simulink model "Pacemaker_Final_01"  (R2020a)
settings: Solver=FixedStepAuto  StartTime=0.0  StopTime=10.0  FixedStep=1e-3  RelTol=1e-3  EnableMultiTasking=on
undefined symbols (not defined in the file): D0, D1, D10, D11, D12, D13, D2, D3, D4, D5, D6, D7, D8, D9, PTA0, PTA1, PTA2, PTB23, PTB9, PTC16, PTC17, PTC2, PTC3, PTC4, PTD0, PTD1, PTD2, PTD3
libraries: frdmk64flib x20
settings Model: ExtModeTrigDuration=5  Creator=forre  LastModifiedBy=forre
settings OptimizationCC: EnhancedBackFolding=on  PassReuseOutputArgsAs=Individual arguments  ZeroExternalMemoryAtStartup=off  ZeroInternalMemoryAtStartup=off  MaxStackSize=64  OptimizeBlockOrder=speed  DifferentSizesBufferReuse=on  OptimizationCustomize=off  EfficientTunableParamExpr=on
settings DebuggingCC: ParameterTunabilityLossMsg=error
settings HardwareCC: ProdBitPerPointer=32  ProdBitPerSizeT=32  ProdBitPerPtrDiffT=32  ProdLargestAtomicInteger=Long  ProdLargestAtomicFloat=Double  ProdWordSize=32  ProdHWDeviceType=ARM Compatible->ARM Cortex
settings SFSimCC: MATLABDynamicMemAlloc=off
settings RTWCC: SystemTargetFile=ert.tlc  HardwareBoard=NXP FRDM-K64F  TemplateMakefile=ert_default_tmf  Toolchain=GNU Tools for ARM Embedded Processors
settings CodeAppCC: ForceParamTrailComments=on  IgnoreCustomStorageClasses=off  OperatorAnnotations=on  SimulinkDataObjDesc=on  SFDataObjDesc=on  InsertBlockDesc=on

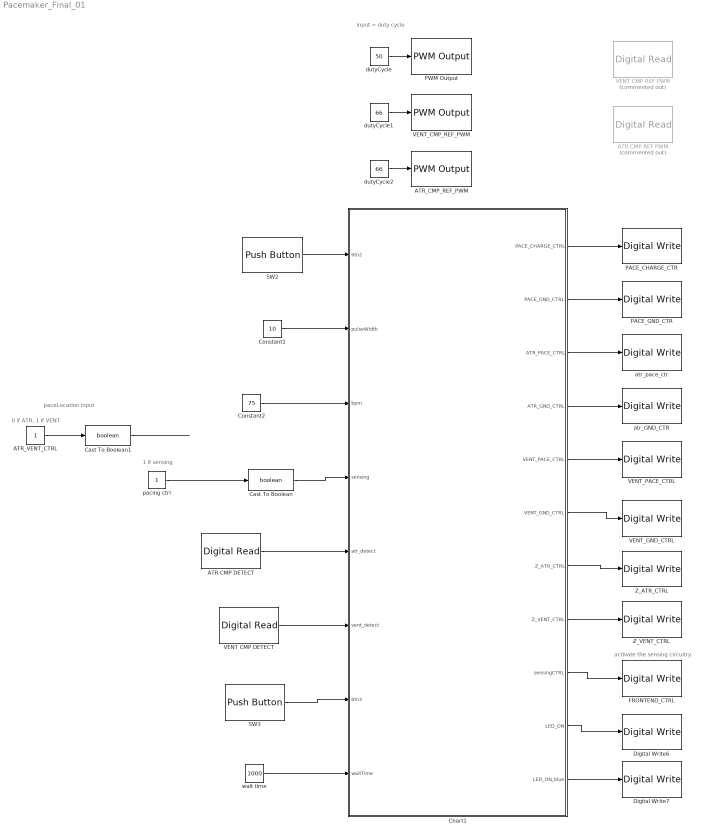
== system Pacemaker_Final_01 ==
  note: paceLocation input
  note: activate the sensing circuitry.
  note: 0 if ATR, 1 if VENT
  note: input = duty cycle
  note: 1 if sensing
  ATR CMP DETECT : frdmk64flib/Digital Read  Whichpin=PTC16 (D0)  SampleTime=-1
  ATR CMP REF PWM : frdmk64flib/Digital Read  Commented=on  Whichpin=PTC2 (D6)  SampleTime=-1
  ATR_CMP_REF_PWM : frdmk64flib/PWM Output  Whichpin=PTC2 (D6)  InitialFrequency=2000  InitialDutyCycle=50
  ATR_VENT_CTRL : Constant
  Cast To Boolean : DataTypeConversion  OutDataTypeStr=boolean
  Cast To Boolean1 : DataTypeConversion  OutDataTypeStr=boolean
  Chart1 : Stateflow chart  TreatAsAtomicUnit=on
  Constant1 : Constant  Value=10
  Constant2 : Constant  Value=75
  Digital Write6 : frdmk64flib/Digital Write  Whichpin=RED_LED
  Digital Write7 : frdmk64flib/Digital Write  Whichpin=BLUE_LED
  FRONTEND_CTRL : frdmk64flib/Digital Write  Whichpin=PTD1 (D13)
  PACE_CHARGE_CTR : frdmk64flib/Digital Write  Whichpin=PTB9 (D2)
  PACE_GND_CTR : frdmk64flib/Digital Write  Whichpin=PTD0 (D10)
  PWM Output : frdmk64flib/PWM Output  Whichpin=PTA2 (D5)  InitialFrequency=2000  InitialDutyCycle=50
  SW2 : frdmk64flib/Push Button  Whichswitch=SW2  SampleTime1=-1
  SW3 : frdmk64flib/Push Button  Whichswitch=SW3  SampleTime1=-1
  VENT CMP DETECT : frdmk64flib/Digital Read  Whichpin=PTC17 (D1)  SampleTime=-1
  VENT CMP REF PWM : frdmk64flib/Digital Read  Commented=on  Whichpin=PTA1 (D3)  SampleTime=-1
  VENT_CMP_REF_PWM : frdmk64flib/PWM Output  Whichpin=PTA1 (D3)  InitialFrequency=2000  InitialDutyCycle=50
  VENT_GND_CTRL : frdmk64flib/Digital Write  Whichpin=PTD3 (D12)
  VENT_PACE_CTRL : frdmk64flib/Digital Write  Whichpin=PTC4 (D9)
  Z_ATR_CTRL : frdmk64flib/Digital Write  Whichpin=PTB23 (D4)
  Z_VENT_CTRL : frdmk64flib/Digital Write  Whichpin=PTC3 (D7)
  atr_GND_CTR : frdmk64flib/Digital Write  Whichpin=PTD2 (D11)
  atr_pace_ctr : frdmk64flib/Digital Write  Whichpin=PTA0 (D8)
  dutyCycle : Constant  Value=50
  dutyCycle1 : Constant  Value=66
  dutyCycle2 : Constant  Value=66
  pacing ctrl : Constant
  wait time : Constant  Value=1000
  wires:
  dutyCycle/1 -> PWM Output/1
  SW2/1 -> Chart1/1(btn2)
  Chart1/4(ATR_GND_CTRL) -> atr_GND_CTR/1
  Constant1/1 -> Chart1/2(pulseWidth)
  Chart1/3(ATR_PACE_CTRL) -> atr_pace_ctr/1
  Chart1/1(PACE_CHARGE_CTRL) -> PACE_CHARGE_CTR/1
  Chart1/2(PACE_GND_CTRL) -> PACE_GND_CTR/1
  Constant2/1 -> Chart1/3(bpm)
  Chart1/5(VENT_PACE_CTRL) -> VENT_PACE_CTRL/1
  Chart1/6(VENT_GND_CTRL) -> VENT_GND_CTRL/1
  Chart1/7(Z_ATR_CTRL) -> Z_ATR_CTRL/1
  Chart1/8(Z_VENT_CTRL) -> Z_VENT_CTRL/1
  ATR_VENT_CTRL/1 -> Cast To Boolean1/1
  pacing ctrl/1 -> Cast To Boolean/1
  ATR CMP DETECT/1 -> Chart1/5(atr_detect)
  VENT CMP DETECT/1 -> Chart1/6(vent_detect)
  dutyCycle1/1 -> VENT_CMP_REF_PWM/1
  dutyCycle2/1 -> ATR_CMP_REF_PWM/1
  Chart1/9(sensingCTRL) -> FRONTEND_CTRL/1
  Cast To Boolean/1 -> Chart1/4(sensing)
  Cast To Boolean1/1 -> ?
  Chart1/10(LED_ON) -> Digital Write6/1
  Chart1/11(LED_ON_blue) -> Digital Write7/1
  SW3/1 -> Chart1/7(btn3)
  wait time/1 -> Chart1/8(waitTime)

== stateflow chart Pacemaker_Final_01/Chart1 ==
  state SENSING_VENT_TRUE
    entry:
    sensingCTRL = true;
  note: VENT PACING
  state VENT_CHARGING_AND_DISCHARGE
    entry:
    PACE_GND_CTRL = true; % 10
    ATR_PACE_CTRL = false;
    Z_VENT_CTRL = false;
    Z_ATR_CTRL = false
    VENT_PACE_CTRL = false;
    VENT_GND_CTRL = true; % 7
    ATR_GND_CTRL = false; % 7
    PACE_CHARGE_CTRL = true;
    secPerBeat = 60/bpm;
    sensingCTRL = sensing;
    %led test
    LED_ON = true;
  state VENT_PACING
    entry:
    PACE_GND_CTRL = true; %10
    VENT_PACE_CTRL = true;
    VENT_GND_CTRL = false; %7
    Z_VENT_CTRL = false;
    Z_ATR_CTRL = false;
    ATR_GND_CTRL = false; %7
    ATR_PACE_CTRL = false; % 6
    sensingCTRL = sensing;
    LED_ON = false;
  state changeLocation1
    entry:
    btn2 == false;
  state changeLocation
    entry:
    btn2 == false;
  note: vent
  note: atr
  note: ATR PACING
  state ATR_CHARGING_AND_DISCHARGE
    entry:
    secPerBeat = 60/bpm;
    sensingCTRL = sensing;
    ATR_PACE_CTRL = false;
    VENT_PACE_CTRL = false;
    PACE_CHARGE_CTRL = true;
    PACE_GND_CTRL = true; % 10
    Z_VENT_CTRL = false;
    Z_ATR_CTRL = false;
    VENT_GND_CTRL = false; % 7
    ATR_GND_CTRL = true; % 7
    %testing
    LED_ON = false;
    LED_ON_blue = false;
  state ATR_PACING
    entry:
    PACE_GND_CTRL = true; %10
    VENT_PACE_CTRL = false;
    VENT_GND_CTRL = false; %7
    Z_VENT_CTRL = false;
    Z_ATR_CTRL = false;
    ATR_GND_CTRL = false; %7
    ATR_PACE_CTRL = true; % 6
    %testing
    LED_ON_blue = true;
  state SENSING_ATR_TRUE
    entry:
    sensingCTRL = true;
  SENSING_VENT_TRUE -> SENSING_VENT_TRUE [order 2] : [sensingCTRL && (vent_detect || btn3)]
  VENT_CHARGING_AND_DISCHARGE -> SENSING_VENT_TRUE [order 3] : [sensingCTRL && (vent_detect || btn3)]
  SENSING_VENT_TRUE -> VENT_CHARGING_AND_DISCHARGE [order 1] : after(waitTime,msec)
  VENT_PACING -> VENT_CHARGING_AND_DISCHARGE : after(pulseWidth, msec)
  VENT_CHARGING_AND_DISCHARGE -> VENT_PACING [order 1] : after(secPerBeat, sec){PACE_CHARGE_CTRL = false;}
  VENT_CHARGING_AND_DISCHARGE -> changeLocation1 [order 4] : [paceLocation==false]
  VENT_CHARGING_AND_DISCHARGE -> VENT_CHARGING_AND_DISCHARGE [order 2] : [btn2]{paceLocation =false}
  ATR_CHARGING_AND_DISCHARGE -> VENT_CHARGING_AND_DISCHARGE [commented out] : [paceLocation==true]
  VENT_CHARGING_AND_DISCHARGE -> ATR_CHARGING_AND_DISCHARGE [commented out] : [paceLocation==false]
  changeLocation -> VENT_CHARGING_AND_DISCHARGE : [true]
  changeLocation1 -> ATR_CHARGING_AND_DISCHARGE : [true]
  ATR_CHARGING_AND_DISCHARGE -> changeLocation [order 4] : [paceLocation==true]
  (default) -> ATR_CHARGING_AND_DISCHARGE
  ATR_CHARGING_AND_DISCHARGE -> ATR_PACING [order 1] : after(secPerBeat, sec){PACE_CHARGE_CTRL = false;}
  ATR_CHARGING_AND_DISCHARGE -> ATR_CHARGING_AND_DISCHARGE [order 2] : [btn2]{paceLocation = true}
  ATR_CHARGING_AND_DISCHARGE -> SENSING_ATR_TRUE [order 3] : [sensingCTRL && (atr_detect || btn3)]
  SENSING_ATR_TRUE -> ATR_CHARGING_AND_DISCHARGE [order 1] : after(waitTime,msec)
  ATR_PACING -> ATR_CHARGING_AND_DISCHARGE : after(pulseWidth, msec)
  SENSING_ATR_TRUE -> SENSING_ATR_TRUE [order 2] : [sensingCTRL && (atr_detect || btn3)]
  data: PACE_CHARGE_CTRL output boolean; PACE_GND_CTRL output boolean; btn2 input boolean; ATR_PACE_CTRL output boolean; ATR_GND_CTRL output boolean; pulseWidth input double; bpm input double; secPerBeat local double; VENT_PACE_CTRL output boolean; VENT_GND_CTRL output boolean; Z_ATR_CTRL output boolean; Z_VENT_CTRL output boolean; sensing input boolean; atr_detect input boolean; vent_detect input boolean; sensingCTRL output boolean; LED_ON output boolean; LED_ON_blue output boolean; paceLocation local boolean; btn3 input boolean; waitTime input double
  data atr_detect settings: description=|
      | 0 = pace atrium
      | 1 = pace ventricle
  data vent_detect settings: description=|
      | 0 = pace atrium
      | 1 = pace ventricle
  data paceLocation settings: description=|
      | 0 = pace atrium
      | 1 = pace ventricle
